simulink model "Final_Simulink_NOV26"  (R2022a)
settings: Solver=VariableStepAuto  StartTime=0.0  StopTime=10.0  RelTol=1e-3
undefined symbols (not defined in the file): D0, D1, D10, D11, D12, D13, D2, D3, D5, D6, D8, D9, PTA0, PTA1, PTA2, PTB9, PTC16, PTC17, PTC2, PTC4, PTD0, PTD1, PTD2, PTD3
libraries: frdmk64flib x17, etargetslib x9
settings Model: Creator=yutousama  LastModifiedBy=jacqu

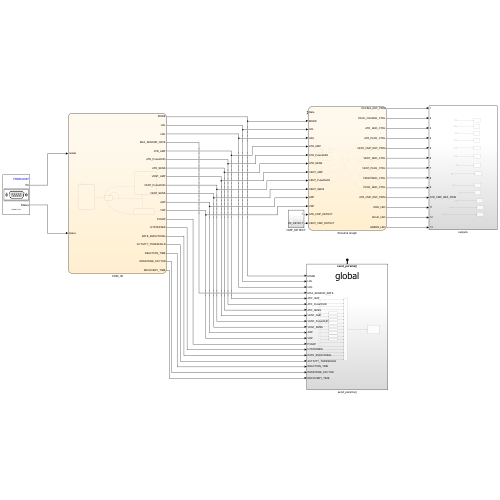
[thumbnail: Simulink's stored preview of the top-level diagram]
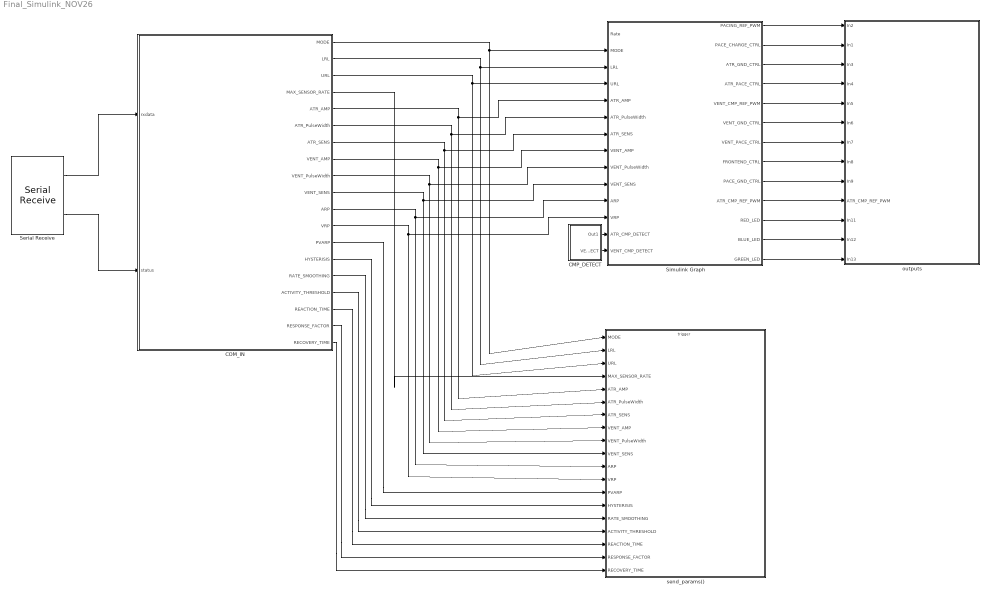
== system Final_Simulink_NOV26 ==
  CMP_DETECT : Subsystem
  COM_IN : Stateflow chart  TreatAsAtomicUnit=on
  Serial Receive : frdmk64flib/Serial Receive  SCIModule=0  Baudrate=uint32(9600)  Parity=None  StopBits=1  HardwareFlowControl=None  ByteOrder=LittleEndian  DataType=uint8  DataLength=42  BlockingMode=off  OutputStatus=on  SampleTime=-1
  Simulink Graph : Stateflow chart  TreatAsAtomicUnit=on
      settings: PortSchema="{\"entries\":[{\"content\":{\"sides\":[{\"content\":{\"connectorIds\":[\"In2\",\"In7\",\"In6\",\"In12\",\"In11\",\"In1\",\"In13\",\"In8\",\"In3\",\"In14\",\"In4\",\"In5\",\"In10\",\"In9\"]},\"type\":\"ConnectorPlacement.EquallySpacedRectSide\",\"uuid\":\"d940ad07-1b63-4409-b611-d8daeaaac01f\"},{\"content\":{\"connectorIds\":[\"Out1\",\"Out2\",\"Out3\",\"Out4\",\"Out5\",\"Out6\",\"Out7\",\"Out8\",\"Out9\",\"Out10\",\"Out11\",\"Out13\",\"Out12\"],\"side\":\"RIGHT\"},\"type\":\"ConnectorPlacement.EquallySpacedRectSide\",\"uuid\":\"31975398-765c-495c-9d3f-31d94c58add8\"},{\"content\":{\"connectorIds\":[],\"side\":\"TOP\"},\"type\":\"ConnectorPlacement.EquallySpacedRectSide\",\"uuid\":\"e476108f-112c-4322-8fc6-7d10629c20a4\"}]},\"type\":\"ConnectorPlacement.EquallySpacedConnector\",\"uuid\":\"855ec6f6-1657-4372-87ad-c48717fb390d\"}],\"packageUris\":[\"http://schema.mathworks.com/mf0/Connector/R2020b\"],\"version\":\"1.0\"}"
  outputs : Subsystem
  send_params() : Subsystem
  wires:
  Simulink Graph/1(PACING_REF_PWM) -> outputs/1(In2)
  Simulink Graph/2(PACE_CHARGE_CTRL) -> outputs/2(In1)
  Simulink Graph/4(ATR_PACE_CTRL) -> outputs/4(In4)
  Simulink Graph/5(VENT_CMP_REF_PWM) -> outputs/5(In5)
  Simulink Graph/6(VENT_GND_CTRL) -> outputs/6(In6)
  Simulink Graph/7(VENT_PACE_CTRL) -> outputs/7(In7)
  Simulink Graph/8(FRONTEND_CTRL) -> outputs/8(In8)
  Simulink Graph/9(PACE_GND_CTRL) -> outputs/9(In9)
  Simulink Graph/13(BLUE_LED) -> outputs/12(In12)
  Simulink Graph/12(GREEN_LED) -> outputs/13(In13)
  Simulink Graph/3(ATR_GND_CTRL) -> outputs/3(In3)
  Simulink Graph/11(RED_LED) -> outputs/11(In11)
  Simulink Graph/10(ATR_CMP_REF_PWM) -> outputs/10(ATR_CMP_REF_PWM)
  Serial Receive/1 -> COM_IN/1(rxdata)
  Serial Receive/2 -> COM_IN/2(status)
  CMP_DETECT/1(Out1) -> Simulink Graph/10(ATR_CMP_DETECT)
  CMP_DETECT/2(VENT_CMP_DETECT) -> Simulink Graph/9(VENT_CMP_DETECT)
  COM_IN/1(MODE) -> Simulink Graph/7(MODE), send_params()/1(MODE)
  COM_IN/2(LRL) -> send_params()/2(LRL), Simulink Graph/6(LRL)
  COM_IN/3(URL) -> send_params()/3(URL), Simulink Graph/12(URL)
  COM_IN/5(ATR_AMP) -> send_params()/5(ATR_AMP), Simulink Graph/11(ATR_AMP)
  COM_IN/6(ATR_PulseWidth) -> send_params()/6(ATR_PulseWidth), Simulink Graph/1(ATR_PulseWidth)
  COM_IN/7(ATR_SENS) -> send_params()/7(ATR_SENS), Simulink Graph/13(ATR_SENS)
  COM_IN/8(VENT_AMP) -> send_params()/8(VENT_AMP), Simulink Graph/8(VENT_AMP)
  COM_IN/9(VENT_PulseWidth) -> send_params()/9(VENT_PulseWidth), Simulink Graph/3(VENT_PulseWidth)
  COM_IN/10(VENT_SENS) -> send_params()/10(VENT_SENS), Simulink Graph/14(VENT_SENS)
  COM_IN/11(ARP) -> send_params()/11(ARP), Simulink Graph/4(ARP)
  COM_IN/12(VRP) -> send_params()/12(VRP), Simulink Graph/5(VRP)
  COM_IN/4(MAX_SENSOR_RATE) -> send_params()/4(MAX_SENSOR_RATE)
  COM_IN/13(PVARP) -> send_params()/13(PVARP)
  COM_IN/14(HYSTERISIS) -> send_params()/14(HYSTERISIS)
  COM_IN/15(RATE_SMOOTHING) -> send_params()/15(RATE_SMOOTHING)
  COM_IN/16(ACTIVITY_THRESHOLD) -> send_params()/16(ACTIVITY_THRESHOLD)
  COM_IN/17(REACTION_TIME) -> send_params()/17(REACTION_TIME)
  COM_IN/18(RESPONSE_FACTOR) -> send_params()/18(RESPONSE_FACTOR)
  COM_IN/19(RECOVERY_TIME) -> send_params()/19(RECOVERY_TIME)

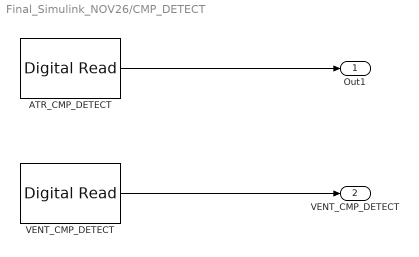
== system Final_Simulink_NOV26/CMP_DETECT ==
  ATR_CMP_DETECT : frdmk64flib/Digital Read  Whichpin=PTC16 (D0)  SampleTime=-1
  "VENT_CMP_DETECT " : frdmk64flib/Digital Read  Whichpin=PTC17 (D1)  SampleTime=-1
  Out1 : Outport
  VENT_CMP_DETECT : Outport  Port=2
  wires:
  "VENT_CMP_DETECT "/1 -> VENT_CMP_DETECT/1
  ATR_CMP_DETECT/1 -> Out1/1

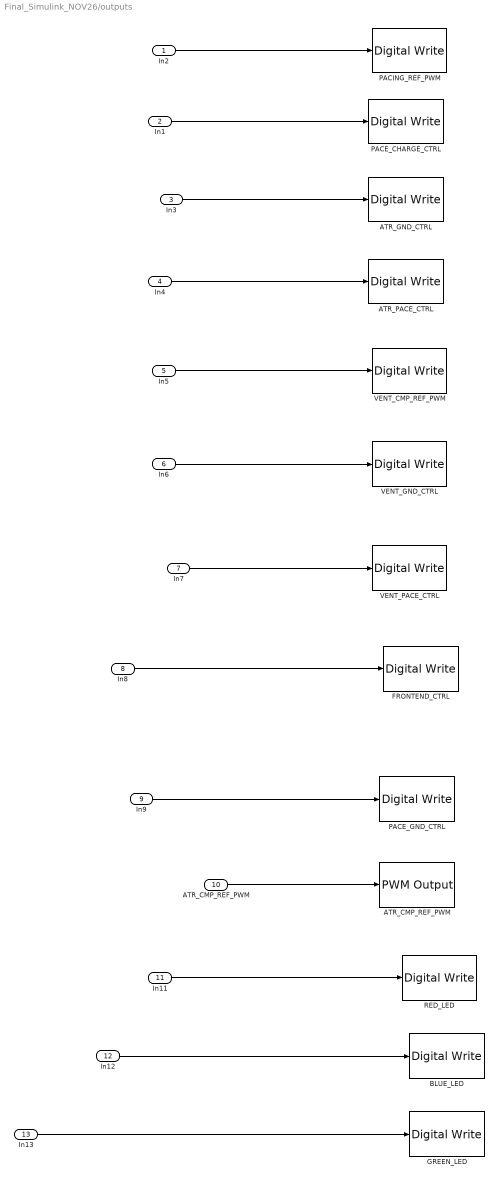
== system Final_Simulink_NOV26/outputs ==
  In2 : Inport
  In1 : Inport  Port=2
  In3 : Inport  Port=3
  In4 : Inport  Port=4
  In5 : Inport  Port=5
  In6 : Inport  Port=6
  In7 : Inport  Port=7
  In8 : Inport  Port=8
  In9 : Inport  Port=9
  ATR_CMP_REF_PWM : Inport  Port=10
  In11 : Inport  Port=11
  In12 : Inport  Port=12
  In13 : Inport  Port=13
  " ATR_CMP_REF_PWM" : frdmk64flib/PWM Output  Whichpin=PTC2 (D6)  InitialFrequency=2000  InitialDutyCycle=0
  ATR_GND_CTRL : frdmk64flib/Digital Write  Whichpin=PTD2 (D11)
  ATR_PACE_CTRL : frdmk64flib/Digital Write  Whichpin=PTA0 (D8)
  BLUE_LED : frdmk64flib/Digital Write  Whichpin=BLUE_LED
  FRONTEND_CTRL : frdmk64flib/Digital Write  Whichpin=PTD1 (D13)
  GREEN_LED : frdmk64flib/Digital Write  Whichpin=GREEN_LED
  PACE_CHARGE_CTRL : frdmk64flib/Digital Write  Whichpin=PTB9 (D2)
  PACE_GND_CTRL : frdmk64flib/Digital Write  Whichpin=PTD0 (D10)
  PACING_REF_PWM : frdmk64flib/Digital Write  Whichpin=PTA2 (D5)
  RED_LED : frdmk64flib/Digital Write  Whichpin=RED_LED
  VENT_CMP_REF_PWM : frdmk64flib/Digital Write  Whichpin=PTA1 (D3)
  VENT_GND_CTRL : frdmk64flib/Digital Write  Whichpin=PTD3 (D12)
  VENT_PACE_CTRL : frdmk64flib/Digital Write  Whichpin=PTC4 (D9)
  wires:
  In2/1 -> PACING_REF_PWM/1
  In1/1 -> PACE_CHARGE_CTRL/1
  In4/1 -> ATR_PACE_CTRL/1
  In5/1 -> VENT_CMP_REF_PWM/1
  In6/1 -> VENT_GND_CTRL/1
  In7/1 -> VENT_PACE_CTRL/1
  In8/1 -> FRONTEND_CTRL/1
  In9/1 -> PACE_GND_CTRL/1
  In12/1 -> BLUE_LED/1
  In13/1 -> GREEN_LED/1
  In11/1 -> RED_LED/1
  In3/1 -> ATR_GND_CTRL/1
  ATR_CMP_REF_PWM/1 -> " ATR_CMP_REF_PWM"/1

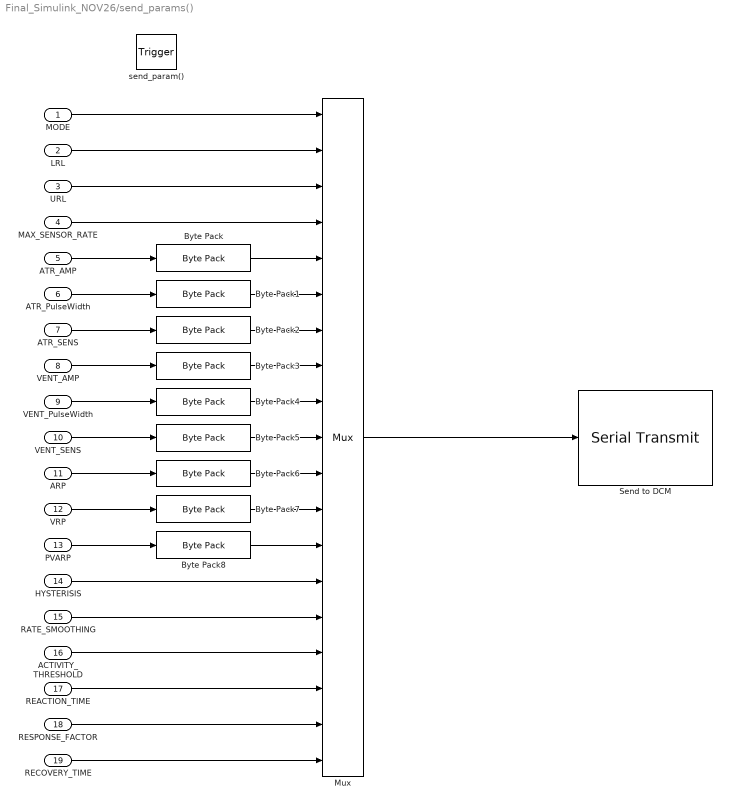
== system Final_Simulink_NOV26/send_params() ==
  MODE : Inport
  LRL : Inport  Port=2
  URL : Inport  Port=3
  MAX_SENSOR_RATE : Inport  Port=4
  ATR_AMP : Inport  Port=5
  ATR_PulseWidth : Inport  Port=6
  ATR_SENS : Inport  Port=7
  VENT_AMP : Inport  Port=8
  VENT_PulseWidth : Inport  Port=9
  VENT_SENS : Inport  Port=10
  ARP : Inport  Port=11
  VRP : Inport  Port=12
  PVARP : Inport  Port=13
  HYSTERISIS : Inport  Port=14
  RATE_SMOOTHING : Inport  Port=15
  ACTIVITY_THRESHOLD : Inport  Port=16
  REACTION_TIME : Inport  Port=17
  RESPONSE_FACTOR : Inport  Port=18
  RECOVERY_TIME : Inport  Port=19
  send_param() : TriggerPort  TriggerType=function-call  IsSimulinkFunction=on  FunctionName=send_params  VariantControl=(inherit)  ZeroCross=off  PortDimensions=1
  Byte Pack{,1..5} (6 alike) : etargetslib/Byte Pack  datatypes={'single'}  byteAlign=1
  Byte Pack6 : etargetslib/Byte Pack  datatypes={'uint16'}  byteAlign=1
  Byte Pack7 : etargetslib/Byte Pack  datatypes={'uint16'}  byteAlign=1
  Byte Pack8 : etargetslib/Byte Pack  datatypes={'uint16'}  byteAlign=1
  Mux : Mux  Inputs=19
  Send to DCM : frdmk64flib/Serial Transmit  SCIModule=0  Baudrate=uint32(9600)  Parity=None  StopBits=1  HardwareFlowControl=None  ByteOrder=LittleEndian  BlockingMode=on  OutputStatus=off
  wires:
  Mux/1 -> Send to DCM/1
  MODE/1 -> Mux/1
  LRL/1 -> Mux/2
  URL/1 -> Mux/3
  MAX_SENSOR_RATE/1 -> Mux/4
  ATR_AMP/1 -> Byte Pack/1
  Byte Pack/1 -> Mux/5
  ATR_PulseWidth/1 -> Byte Pack1/1
  Byte Pack1/1 -> Mux/6
  ATR_SENS/1 -> Byte Pack2/1
  Byte Pack2/1 -> Mux/7
  VENT_AMP/1 -> Byte Pack3/1
  Byte Pack3/1 -> Mux/8
  VENT_PulseWidth/1 -> Byte Pack4/1
  Byte Pack4/1 -> Mux/9
  VENT_SENS/1 -> Byte Pack5/1
  Byte Pack5/1 -> Mux/10
  ARP/1 -> Byte Pack6/1
  Byte Pack6/1 -> Mux/11
  VRP/1 -> Byte Pack7/1
  Byte Pack7/1 -> Mux/12
  PVARP/1 -> Byte Pack8/1
  Byte Pack8/1 -> Mux/13
  HYSTERISIS/1 -> Mux/14
  RATE_SMOOTHING/1 -> Mux/15
  ACTIVITY_THRESHOLD/1 -> Mux/16
  REACTION_TIME/1 -> Mux/17
  RESPONSE_FACTOR/1 -> Mux/18
  RECOVERY_TIME/1 -> Mux/19

== stateflow chart Final_Simulink_NOV26/COM_IN ==
  settings: executeAtInitialization=1
  state SET_PARAM
    entry:
    MODE = rxdata(3);
    LRL =  rxdata(4);
    URL = rxdata(5);
    MAX_SENSOR_RATE = rxdata(6);
    ATR_AMP = typecast(rxdata(7:10), 'single');
    ATR_PulseWidth = typecast(rxdata(11:14), 'single');
    ATR_SENS = typecast(rxdata(15:18), 'single');
    VENT_AMP = typecast(rxdata(19:22), 'single');
    VENT_PulseWidth = typecast(rxdata(23:26), 'single');
    VENT_SENS = typecast(rxdata(27:30), 'single');
    ARP = typecast(rxdata(31:32), 'uint16');
    VRP = typecast(rxdata(33:34), 'uint16');
    PVARP = typecast(rxdata(35:36), 'uint16');
    HYSTERISIS = rxdata(37);
    RATE_SMOOTHING = rxdata(38);
    ACTIVITY_THRESHOLD = rxdata(39);
    REACTION_TIME = rxdata(40);
    RESPONSE_FACTOR = rxdata(41);
    RECOVERY_TIME = rxdata(42);
  state INITIAL
    entry:
    MODE = 1;
    LRL =  30;
    URL = 50;
    MAX_SENSOR_RATE = 50;
    ATR_AMP = 0.5;
    ATR_PulseWidth = 0.05;
    ATR_SENS = 0.25;
    VENT_AMP = 0.5;
    VENT_PulseWidth = 0.05;
    VENT_SENS = 0.25;
    ARP = 150;
    VRP = 150;
    PVARP = 150;
    HYSTERISIS = 0;
    RATE_SMOOTHING = 0;
    ACTIVITY_THRESHOLD = 1;
    REACTION_TIME = 10;
    RESPONSE_FACTOR = 1;
    RECOVERY_TIME = 2;
  state STANDBY
    % waiting for COM
  state ECHO_PARAM
    entry:
    send_params();
  (default) -> INITIAL
  SET_PARAM -> STANDBY
  (junction 31) -> STANDBY [order 2]
  (junction 33) -> SET_PARAM [order 1] : [rxdata(2) == hex2dec('55')]
  INITIAL -> STANDBY
  STANDBY -> (junction 31) : [status == 0]
  (junction 31) -> (junction 33) [order 1] : [rxdata(1) == hex2dec('16')]
  (junction 33) -> ECHO_PARAM [order 2] : [rxdata(2) == hex2dec('22')]
  ECHO_PARAM -> STANDBY
  data: rxdata input; status input; MODE output; LRL output; URL output; MAX_SENSOR_RATE output; ATR_AMP output; ATR_PulseWidth output; ATR_SENS output; VENT_AMP output; VENT_PulseWidth output; VENT_SENS output; ARP output; VRP output; PVARP output; HYSTERISIS output; RATE_SMOOTHING output; ACTIVITY_THRESHOLD output; REACTION_TIME output; RESPONSE_FACTOR output; RECOVERY_TIME output

== stateflow chart Final_Simulink_NOV26/Simulink Graph ==
  state AAI_PACE_OFF
    entry:
    ATR_PACE_CTRL = 0
    VENT_PACE_CTRL = 0
    PACING_REF_PWM = ATR_AMP/5*100
    PACE_CHARGE_CTRL = 1
    PACE_GND_CTRL = 1
    ATR_GND_CTRL = 1
    VENT_GND_CTRL = 0
    FRONTEND_CTRL = 1
    ATR_CMP_REF_PWM = ATR_SENS/5*100
    % light indicators
    RED_LED = 0
    GREEN_LED = 0
  state AAI_PACE_ON
    entry:
    PACE_CHARGE_CTRL = 0
    PACE_GND_CTRL = 1
    ATR_PACE_CTRL = 1
    ATR_GND_CTRL = 0
    VENT_GND_CTRL = 0
    VENT_PACE_CTRL = 0
    % light indicator
    RED_LED = 1
  note: at paceon state, the system waits for the atr_cmp_detect signal to decide which
      | mode to go to . if atr_cmp_detect == 0, pace on. else, go refractory mode.
  state AAI_REFRACTORY
    entry:
    FRONTEND_CTRL = 0
    ATR_PACE_CTRL = 0
    ATR_GND_CTRL = 1
    PACING_REF_PWM = ATR_AMP/5*100
    PACE_CHARGE_CTRL = 0
    PACE_GND_CTRL = 1
    % light indicator
    GREEN_LED = 1
    %Atrium Refractory Period
  state AOO
    entry:
    ATR_PACE_CTRL = 0
    VENT_PACE_CTRL = 0
    PACING_REF_PWM = ATR_AMP/5*100
    PACE_CHARGE_CTRL = 1
    PACE_GND_CTRL = 1
    VENT_PACE_CTRL = 0
    ATR_PACE_CTRL = 0
    ATR_GND_CTRL = 1
    VENT_GND_CTRL = 0
    RED_LED = 0
  state PACING_AOO
    entry:
    PACE_CHARGE_CTRL = 0
    PACE_GND_CTRL = 1
    ATR_PACE_CTRL = 1
    ATR_GND_CTRL = 0
    VENT_GND_CTRL = 0
    VENT_PACE_CTRL = 0
    RED_LED = 1
  note: when pacing, after the pulse width,
      | the mode would change to refractory mdoe
  state AOOR
    entry:
    ATR_PACE_CTRL = 0
    VENT_PACE_CTRL = 0
    PACING_REF_PWM = ATR_AMP/5*100
    PACE_CHARGE_CTRL = 1
    PACE_GND_CTRL = 1
    VENT_PACE_CTRL = 0
    ATR_PACE_CTRL = 0
    ATR_GND_CTRL = 1
    VENT_GND_CTRL = 0
    RED_LED = 0
  state PACING_AOOR
    entry:
    PACE_CHARGE_CTRL = 0
    PACE_GND_CTRL = 1
    ATR_PACE_CTRL = 1
    ATR_GND_CTRL = 0
    VENT_GND_CTRL = 0
    VENT_PACE_CTRL = 0
    RED_LED = 1
  state AAIR_PACE_OFF
    entry:
    ATR_PACE_CTRL = 0
    VENT_PACE_CTRL = 0
    PACING_REF_PWM = ATR_AMP/5*100
    PACE_CHARGE_CTRL = 1
    PACE_GND_CTRL = 1
    ATR_GND_CTRL = 1
    VENT_GND_CTRL = 0
    FRONTEND_CTRL = 1
    ATR_CMP_REF_PWM = ATR_SENS/5*100
    % light indicators
    RED_LED = 0
    GREEN_LED = 0
  state AAIR_PACE_ON
    entry:
    PACE_CHARGE_CTRL = 0
    PACE_GND_CTRL = 1
    ATR_PACE_CTRL = 1
    ATR_GND_CTRL = 0
    VENT_GND_CTRL = 0
    VENT_PACE_CTRL = 0
    % light indicator
    RED_LED = 1
  note: at paceon state, the system waits for the atr_cmp_detect signal to decide which
      | mode to go to . if atr_cmp_detect == 0, pace on. else, go refractory mode.
  state INITIAL_INPUTS
    %MODE:
    %1: AOO  2: AOOR  3:VOO  4: VOOR 5: AAI  6:AAIR 7:VVI 8: VVIR
  state AAIR_REFRACTORY
    entry:
    FRONTEND_CTRL = 0
    ATR_PACE_CTRL = 0
    ATR_GND_CTRL = 1
    PACING_REF_PWM = ATR_AMP/5*100
    PACE_CHARGE_CTRL = 0
    PACE_GND_CTRL = 1
    % light indicator
    GREEN_LED = 1
    %Atrium Refractory Period
  note: when pacing, after the pulse width,
      | the mode would change to refractory mdoe
  state VOO
    entry:
    ATR_PACE_CTRL = 0
    VENT_PACE_CTRL = 0
    PACING_REF_PWM = VENT_AMP/5*100
    PACE_CHARGE_CTRL = 1
    PACE_GND_CTRL = 1
    VENT_PACE_CTRL = 0
    ATR_PACE_CTRL = 0
    ATR_GND_CTRL = 0
    VENT_GND_CTRL = 1
    BLUE_LED = 0
  state PACING_VOO
    entry:
    PACE_CHARGE_CTRL = 0
    PACE_GND_CTRL = 1
    ATR_PACE_CTRL = 0
    ATR_GND_CTRL = 0
    VENT_GND_CTRL = 0
    VENT_PACE_CTRL = 1
    BLUE_LED = 1
  state VVI_PACE_OFF
    entry:
    ATR_PACE_CTRL = 0
    VENT_PACE_CTRL = 0
    PACING_REF_PWM = VENT_AMP/5*100
    PACE_CHARGE_CTRL = 1
    PACE_GND_CTRL = 1
    VENT_PACE_CTRL = 0
    ATR_PACE_CTRL = 0
    ATR_GND_CTRL = 1
    VENT_GND_CTRL = 0
    FRONTEND_CTRL = 1
    VENT_CMP_REF_PWM = VENT_SENS/5*100
    % light indicators
    BLUE_LED = 0
    GREEN_LED = 0
  state VVI_PACE_ON
    entry:
    PACE_CHARGE_CTRL = 0
    PACE_GND_CTRL = 1
    ATR_PACE_CTRL = 0
    ATR_GND_CTRL = 0
    VENT_GND_CTRL = 0
    VENT_PACE_CTRL = 1
    % light indicator
    BLUE_LED = 1
  note: at pace_off state and wait for the vent_cmp_detect signal to decide which
      | mode to go to.
  note: vent_cmp_detect = 1, the heart works fine, so refractory mode
  state VVI_REFRACTORY
    entry:
    FRONTEND_CTRL = 0
    VENT_PACE_CTRL = 0
    VENT_GND_CTRL = 1
    PACING_REF_PWM = VENT_AMP/5*100
    PACE_CHARGE_CTRL = 0
    PACE_GND_CTRL = 1
    % light indicator
    GREEN_LED = 1
  state VOOR
    entry:
    ATR_PACE_CTRL = 0
    VENT_PACE_CTRL = 0
    PACING_REF_PWM = VENT_AMP/5*100
    PACE_CHARGE_CTRL = 1
    PACE_GND_CTRL = 1
    VENT_PACE_CTRL = 0
    ATR_PACE_CTRL = 0
    ATR_GND_CTRL = 0
    VENT_GND_CTRL = 1
    BLUE_LED = 0
  state PACING_VOOR
    entry:
    PACE_CHARGE_CTRL = 0
    PACE_GND_CTRL = 1
    ATR_PACE_CTRL = 0
    ATR_GND_CTRL = 0
    VENT_GND_CTRL = 0
    VENT_PACE_CTRL = 1
    BLUE_LED = 1
  state VVIR_PACE_OFF
    entry:
    ATR_PACE_CTRL = 0
    VENT_PACE_CTRL = 0
    PACING_REF_PWM = VENT_AMP/5*100
    PACE_CHARGE_CTRL = 1
    PACE_GND_CTRL = 1
    VENT_PACE_CTRL = 0
    ATR_PACE_CTRL = 0
    ATR_GND_CTRL = 1
    VENT_GND_CTRL = 0
    FRONTEND_CTRL = 1
    VENT_CMP_REF_PWM = VENT_SENS/5*100
    % light indicators
    BLUE_LED = 0
    GREEN_LED = 0
  state VVIR_PACE_ON
    entry:
    PACE_CHARGE_CTRL = 0
    PACE_GND_CTRL = 1
    ATR_PACE_CTRL = 0
    ATR_GND_CTRL = 0
    VENT_GND_CTRL = 0
    VENT_PACE_CTRL = 1
    % light indicator
    BLUE_LED = 1
  note: at pace_off state and wait for the vent_cmp_detect signal to decide which
      | mode to go to.
  note: vent_cmp_detect = 1, the heart works fine, so refractory mode
  state VVIR_REFRACTORY
    entry:
    FRONTEND_CTRL = 0
    VENT_PACE_CTRL = 0
    VENT_GND_CTRL = 1
    PACING_REF_PWM = VENT_AMP/5*100
    PACE_CHARGE_CTRL = 0
    PACE_GND_CTRL = 1
    % light indicator
    GREEN_LED = 1
  AAI_PACE_OFF -> AAI_PACE_ON [order 1] : [(ATR_CMP_DETECT == 0) && after((60000/LRL)-ATR_PulseWidth-ARP,msec)]
  INITIAL_INPUTS -> AOO [order 1] : [MODE == 1]
  INITIAL_INPUTS -> AAI_PACE_OFF [order 5] : [MODE == 5]
  AAI_PACE_ON -> AAI_REFRACTORY : [after(ATR_PulseWidth,msec)]
  AAI_REFRACTORY -> AAI_PACE_OFF : [after(ARP,msec)]
  AAI_PACE_OFF -> AAI_REFRACTORY [order 2] : [ATR_CMP_DETECT == 1]
  AOO -> PACING_AOO : [after((60000/LRL)-ATR_PulseWidth,msec)]
  PACING_AOO -> AOO : [after(ATR_PulseWidth,msec)]
  (default) -> INITIAL_INPUTS
  AOOR -> PACING_AOOR : [after((60000/Rate)-ATR_PulseWidth,msec)]
  INITIAL_INPUTS -> AAIR_PACE_OFF [order 6] : [MODE == 6]
  AAIR_PACE_OFF -> AAIR_PACE_ON [order 1] : [(ATR_CMP_DETECT == 0) && after((60000/Rate)-ATR_PulseWidth-ARP,msec)]
  PACING_AOOR -> AOOR : [after(ATR_PulseWidth,msec)]
  INITIAL_INPUTS -> VVI_PACE_OFF [order 7] : [MODE == 7]
  INITIAL_INPUTS -> AOOR [order 2] : [MODE==2]
  AAIR_PACE_ON -> AAIR_REFRACTORY : [after(ATR_PulseWidth,msec)]
  AAIR_REFRACTORY -> AAIR_PACE_OFF : [after(ARP,msec)]
  AAIR_PACE_OFF -> AAIR_REFRACTORY [order 2] : [ATR_CMP_DETECT == 1]
  INITIAL_INPUTS -> VOO [order 3] : [MODE == 3]
  INITIAL_INPUTS -> VOOR [order 4] : [MODE == 4]
  INITIAL_INPUTS -> VVIR_PACE_OFF [order 8] : [MODE == 8]
  VOO -> PACING_VOO : [after((60000/LRL)-VENT_PulseWidth,msec)]
  PACING_VOO -> VOO : [after(VENT_PulseWidth,msec)]
  VVI_PACE_OFF -> VVI_PACE_ON [order 1] : [(VENT_CMP_DETECT == 0) & after((60000/LRL)-VENT_PulseWidth-VRP,msec)]
  VVI_PACE_ON -> VVI_REFRACTORY : [after(VENT_PulseWidth,msec)]
  VVI_REFRACTORY -> VVI_PACE_OFF : [after(VRP,msec)]
  VVI_PACE_OFF -> VVI_REFRACTORY [order 2] : [VENT_CMP_DETECT == 1]
  VOOR -> PACING_VOOR : [after((60000/Rate)-VENT_PulseWidth,msec)]
  PACING_VOOR -> VOOR : [after(VENT_PulseWidth,msec)]
  VVIR_PACE_OFF -> VVIR_PACE_ON [order 1] : [(VENT_CMP_DETECT == 0) & after((60000/Rate)-VENT_PulseWidth-VRP,msec)]
  VVIR_PACE_ON -> VVIR_REFRACTORY : [after(VENT_PulseWidth,msec)]
  VVIR_REFRACTORY -> VVIR_PACE_OFF : [after(VRP,msec)]
  VVIR_PACE_OFF -> VVIR_REFRACTORY [order 2] : [VENT_CMP_DETECT == 1]
  data: ATR_PulseWidth input; Rate input; VENT_PulseWidth input; PACING_REF_PWM output; PACE_CHARGE_CTRL output; ATR_GND_CTRL output; ATR_PACE_CTRL output; VENT_CMP_REF_PWM output; VENT_GND_CTRL output; VENT_PACE_CTRL output; FRONTEND_CTRL output; PACE_GND_CTRL output; ATR_CMP_REF_PWM output; ARP input; VRP input; LRL input; MODE input; VENT_AMP input; VENT_CMP_DETECT input; ATR_CMP_DETECT input; ATR_AMP input; RED_LED output; GREEN_LED output; URL input; BLUE_LED output; ATR_SENS input; VENT_SENS input
